simulink model "File6"  (Simulink 9.1)
settings: Solver=VariableStepAuto  StartTime=0.0  StopTime=2  RelTol=1e-3
libraries: powerlib x12, powerlib_meascontrol x4, re_lib x1, simulink x1
settings Model: Creator=asus  LastModifiedBy=asus
settings SolverCC: ZeroCrossAlgorithm=Adaptive
settings DataIOCC: SaveFormat=Dataset
settings OptimizationCC: LifeSpan=auto
settings DebuggingCC: UnderspecifiedInitializationDetection=Simplified  MergeDetectMultiDrivingBlocksExec=error  MaxConsecutiveZCsMsg=none  SFUnexpectedBacktrackingDiag=error  SFNoUnconditionalDefaultTransitionDiag=error  SFExecutionAtInitializationDiag=warning
settings HardwareCC: ProdBitPerPointer=64  ProdBitPerSizeT=64  ProdBitPerPtrDiffT=64  ProdLargestAtomicFloat=Float  ProdIntDivRoundTo=Zero  ProdEndianess=LittleEndian  ProdWordSize=64  ProdHWDeviceType=Intel->x86-64 (Windows64)
settings ModelReferenceCC: PropagateSignalLabelsOutOfModel=on
settings CodeAppCC: StateflowObjectComments=off
settings GRTTargetCC: TargetLangStandard=C99 (ISO)  CombineOutputUpdateFcns=on  GRTInterface=off
settings ConfigComp: CovMetricSettings=dwe  CovHtmlReporting=off  CovSaveCumulativeToWorkspaceVar=off  CovSaveSingleToWorkspaceVar=off  CovExternalEMLEnable=on

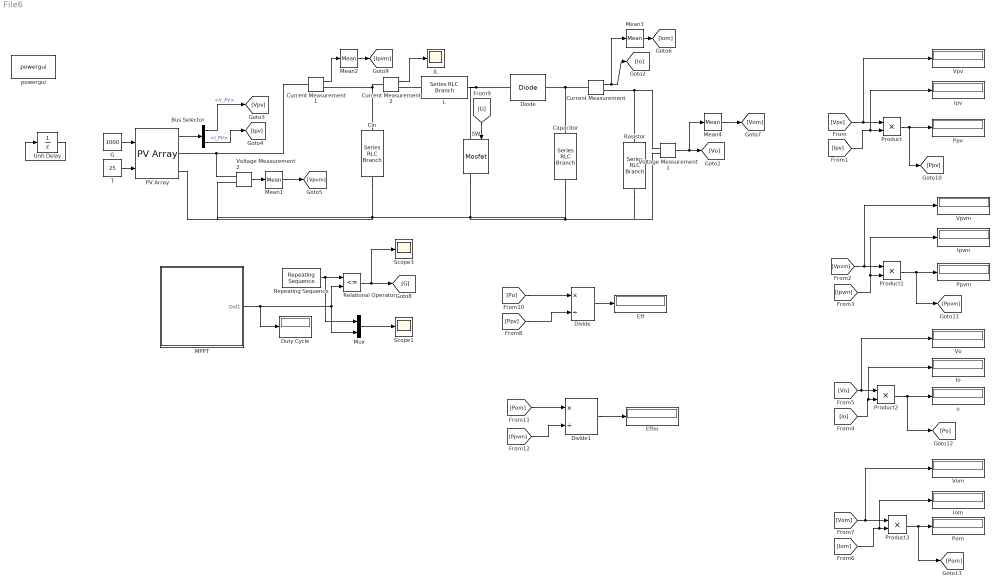
== system File6 ==
  Bus Selector : BusSelector  OutputSignals=V_PV,I_PV
  Capacitor : powerlib/Elements/Series RLC Branch  LConnTagsString=__new0  RConnTagsString=__new0  BranchType=C  Resistance=1  Inductance=1e-3  SetiL0=off  InitialCurrent=0  Capacitance=31.26e-6  Setx0=off  InitialVoltage=0  Measurements=None
  Cin : powerlib/Elements/Series RLC Branch  LConnTagsString=__new0  RConnTagsString=__new0  BranchType=C  Resistance=1  Inductance=583.4e-6  SetiL0=off  InitialCurrent=0  Capacitance=143e-6  Setx0=off  InitialVoltage=0  Measurements=None
  Current Measurement : powerlib/Measurements/Current Measurement  PhasorSimulation=off  OutputType=Complex  PSBequivalent=0
  Current Measurement1 : powerlib/Measurements/Current Measurement  PhasorSimulation=off  OutputType=Complex  PSBequivalent=0
  Current Measurement2 : powerlib/Measurements/Current Measurement  PhasorSimulation=off  OutputType=Complex  PSBequivalent=0
  Diode : powerlib/Power Electronics/Diode  Ron=0.001  Lon=0  Vf=0.8  IC=0  UseSnubber=0  Rs=500  Cs=250e-9  Measurements=off
  Divide : Product  Inputs=*/
  Divide1 : Product  Inputs=*/
  "Duty Cycle " : Display
  Eff : Display
  Effm : Display
  G : Constant  Value=1000
  IL : Scope
  Io : Display
  Iom : Display
  Ipv : Display
  Ipvm : Display
  L : powerlib/Elements/Series RLC Branch  LConnTagsString=__new0  RConnTagsString=__new0  BranchType=L  Resistance=1  Inductance=583.4e-6  SetiL0=off  InitialCurrent=0  Capacitance=1e-6  Setx0=off  InitialVoltage=0  Measurements=None
  MPPT : Subsystem
  Mean{1..4} (4 alike) : powerlib_meascontrol/Measurements/Mean  Freq=60  Vinit=0  Ts=0
  Mux : Mux  Inputs=2
  PV Array : re_lib/Solar/PV Array  Npar=1  Nser=6  PlotType=array @ 1000 W/m2 & specified temperatures  S_vec="[ 1000  500  100 ]"  Temp_C_vec="[ 45 25  ]"  ModuleName=User-defined  PlotWhenSelected=off  Pm=249.9945  Ncell=60  Voc=36.54  Isc=9.44  Vm=30.45  Im=8.21  beta_Voc_pc=-0.32  alpha_Isc_pc=0.04  beta_Voc=-0.11693  alpha_Isc=0.003776  IL=9.4926  I0=6.8452e-11  nI=0.92814  Rsh=34.9757  Rs=0.19485  BAL=off  Tc=1e-6  Tfilter=5e-5
  Pom : Display
  Ppv : Display
  Ppvm : Display
  Product{,1..3} (4 alike) : Product
  Rasistor : powerlib/Elements/Series RLC Branch  LConnTagsString=__new0  RConnTagsString=__new0  BranchType=R  Resistance=70.41  Inductance=1e-3  SetiL0=off  InitialCurrent=0  Capacitance=1e-6  Setx0=off  InitialVoltage=0  Measurements=None
  Relational Operator : RelationalOperator  Operator=<=  OutDataTypeStr=boolean  RndMeth=Simplest
  Repeating Sequence : simulink/Sources/Repeating Sequence  rep_seq_t=[0 2.5e-5 5e-5 7.5e-5 1e-4]  rep_seq_y=[0 325 0 -325 0 ]
  SW : powerlib/Power Electronics/Mosfet  Ron=0.1  Lon=0  Rd=0.01  Vfd=0  IC=0  Rs=1e5  Cs=inf  Measurements=on
  Scope1 : Scope
  Scope3 : Scope
  T : Constant  Value=25
  Unit Delay : UnitDelay  SampleTime=0.000001
  Vo : Display
  Voltage Measurement1 : powerlib/Measurements/Voltage Measurement  PhasorSimulation=off  OutputType=Complex  PSBequivalent=0
  Voltage Measurement2 : powerlib/Measurements/Voltage Measurement  PhasorSimulation=off  OutputType=Complex  PSBequivalent=0
  Vom : Display
  Vpv : Display
  Vpvm : Display
  o : Display
  powergui : powerlib/powergui  Priority=1  SimulationMode=Continuous  SampleTime=1e-6  frequency=60  Iterations=50  frequencyindice=0  Pbase=100e6  ErrMax=1e-4  UnitsV=kV  UnitsW=MW  buscounter=0  FunctionMessages=off  echomessages=off  EnableUseOfTLC=off  CurrentSourceSwitches=off  DisableSnubberDevices=off  DisableRonSwitches=off  DisableVfSwitches=off  DisplayEquations=off  SolverType=Tustin/Backward Euler (TBE)  Interpol=off  ExternalGateDelay=off  methode=off  Ts=100  x0status=blocks  SPID=on  SwTol=0  HookPort=off  RestoreLinks=warning  ResistiveCurrentMeasurement=off  Frange=[0:2:500]  Ylog=off  Xlog=on  ShowGrid=off  save=off  variable=ZData  structure=0  ZoomFFT=off  StartTime=0.0  cycles=1  DisplayStyle=1  fundamental=60  FreqAxis=off  MaxFrequency=1000  frequencyindicesteady=1  RmsSteady=1  display=off
  wires:
  Voltage Measurement1/1 -> Mean4/1, [Vo]
  Current Measurement/1 -> [Io], Mean3/1
  G/1 -> PV Array/1
  T/1 -> PV Array/2
  PV Array/1 -> Bus Selector/1
  Bus Selector/2 -> [Ipv]  "<I_PV>"
  Bus Selector/1 -> [Vpv]  "<V_PV>"
  Voltage Measurement2/1 -> Mean1/1
  Current Measurement1/1 -> Mean2/1
  Mean1/1 -> [Vpvm]
  Mean2/1 -> [Ipvm]
  MPPT/1(Out1) -> Mux/2, Relational Operator/2, "Duty Cycle "/1
  Mean3/1 -> [Iom]
  Mean4/1 -> [Vom]
  Repeating Sequence/1 -> Mux/1, Relational Operator/1
  Relational Operator/1 -> Scope3/1, [G]
  [G] -> SW/1
  Mux/1 -> Scope1/1
  [Vpv] -> Vpv/1, Product/1
  [Ipv] -> Ipv/1, Product/2
  [Vpvm] -> Vpvm/1, Product1/1
  [Ipvm] -> Ipvm/1, Product1/2
  [Vo] -> Vo/1, Product2/1
  [Io] -> Io/1, Product2/2
  [Vom] -> Vom/1, Product3/1
  [Iom] -> Iom/1, Product3/2
  Product/1 -> [Ppv], Ppv/1
  Product1/1 -> [Ppvm], Ppvm/1
  Product2/1 -> [Po], o/1
  Product3/1 -> [Pom], Pom/1
  [Po] -> Divide/1
  [Ppv] -> Divide/2
  [Pom] -> Divide1/1
  [Ppvm] -> Divide1/2
  Divide/1 -> Eff/1
  Divide1/1 -> Effm/1
  Current Measurement2/1 -> IL/1
  Unit Delay/1 -> Unit Delay/1
  connections:
  PV Array/RConn1 -- Current Measurement1/LConn1 -- Voltage Measurement2/LConn1
  L/RConn1 -- SW/LConn1 -- Diode/LConn1
  SW/RConn1 -- Voltage Measurement1/LConn2 -- Rasistor/RConn1 -- Capacitor/RConn1 -- Voltage Measurement2/LConn2 -- PV Array/RConn2 -- Cin/RConn1
  Capacitor/LConn1 -- Current Measurement/LConn1 -- Diode/RConn1
  Rasistor/LConn1 -- Voltage Measurement1/LConn1 -- Current Measurement/RConn1
  Cin/LConn1 -- Current Measurement2/LConn1 -- Current Measurement1/RConn1
  L/LConn1 -- Current Measurement2/RConn1

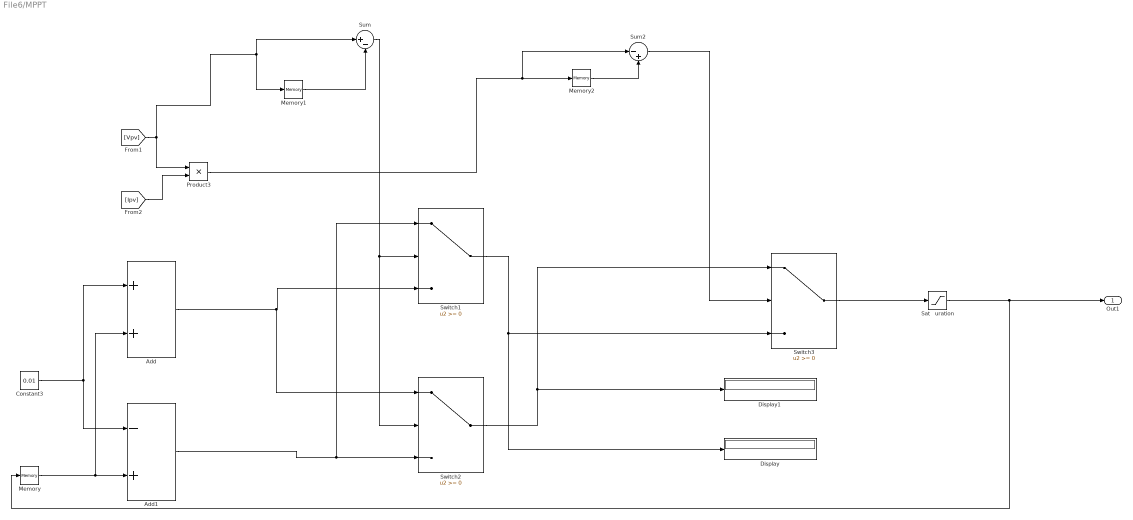
== system File6/MPPT ==
  Add : Sum
  Add1 : Sum  Inputs=-+
  Constant3 : Constant  Value=0.01
  Display : Display
  Display1 : Display
  Memory : Memory
  Memory1 : Memory
  Memory2 : Memory
  Product3 : Product
  Sat   uration : Saturate  UpperLimit=1  LowerLimit=-1
  Sum : Sum  Inputs=|+-
  Sum2 : Sum  Inputs=|-+
  Switch1 : Switch
  Switch2 : Switch
  Switch3 : Switch
  Out1 : Outport
  wires:
  [Vpv] -> Memory1/1, Sum/1, Product3/1
  Constant3/1 -> Add/1, Add1/1
  [Ipv] -> Product3/2
  Add1/1 -> Switch1/1, Switch2/3
  Sum2/1 -> Switch3/2
  Switch1/1 -> Switch3/3, Display/1
  Sat   uration/1 -> Memory/1, Out1/1
  Add/1 -> Switch2/1, Switch1/3
  Memory/1 -> Add/2, Add1/2
  Switch3/1 -> Sat   uration/1
  Switch2/1 -> Display1/1, Switch3/1
  Product3/1 -> Sum2/1, Memory2/1
  Memory1/1 -> Sum/2
  Sum/1 -> Switch1/2, Switch2/2
  Memory2/1 -> Sum2/2
